simulink model "hybrid_lht_accumulator"  (R2019b)
settings: Solver=FixedStepDiscrete  StartTime=0.0  StopTime=inf  FixedStep=1/150e6  RelTol=1e-3
InitFcn:
  | hybrid_lht_setup;
StopFcn:
  | hybrid_lht_accumulator_compare;
undefined symbols (not defined in the file or in its folder): bt, height, nTheta, width
libraries: hdlsllib x20, simulink x17, dspsrcs4 x1
(part 2 of 2)

== system hybrid_lht_accumulator/Hybrid LHT/Hybrid LHT Accumulator/Accumulator with Switches/Accumulator/Block RAM ==
  wr_data : Inport
  wr_addr : Inport  Port=2
  wr_en : Inport  Port=3
  rd_addr : Inport  Port=4
  Simple Dual Port RAM : Subsystem  VariantControl=9_bits
  Simple Dual Port RAM Generator : Subsystem  VariantControl=other_bits  mask{b=36, d=400, b_hidden=12, d_hidden=2204}
      mask prompts: b "Data width:"; d "Depth:"
      mask init:
      | if b == b_hidden && d == d_hidden
      |     return
      | end
      | 
      | % Xilinx RAM Initialisation
      | xl_config = [512, 72;
      |             1024, 36;
      |             2048, 18;
      |             4096, 9;
      |             8192, 4;
      |             16384, 2;
      |             32768, 1];
      | 
      | % Get length of Xilinx Configuration
      | sizeram = size(xl_config);
      |         
      | % Get the RAM Configuration based on the data width
      | for i = 1:sizeram(1)
      |     if b <= xl_config(i, 2)
      |         a = xl_config(i, :);
      |     end
      | end
      | 
      | % Get number of BRAM required (including half BRAM)
      | numbram = ceil((d/a(1))/0.5)*0.5;
      | fullbram = floor(numbram); % Integer
      | halfbram = (numbram-floor(numbram)) ~= 0; % Boolean
      | 
      | % Get all blocks and delete everything excepts ports
      | H = get(find_system(gcb, 'FindAll', 'on', 'type', 'block'));
      | todelete = setdiff(strcat(repmat({[gcb '/']}, numel(H.Blocks), 1),  H.Blocks),...
      |     strcat(repmat({[gcb '/']}, 5, 1),...
      |     {'wr_data'; 'wr_addr'; 'wr_en'; 'rd_addr'; 'rd_data'}));
      | delete_block(todelete);
      | 
      | % Delete lines
      | for i = 1:numel(H.Lines)
      |     delete_line(H.Lines(i).Handle)
      | end
      | 
      | % Generate full BRAMs
      | y = 0;
      | 
      | % If there is only one ram then the write enable should be directly
      | % connected to the first ram write enable. Else, the write address must be sliced
      | % and the upper bound (over a(2)) compared to zero. This will indicate if
      | % the first ram is the one to be written/read from.
      | 
      | % Common to both implementations
      | % Write Address Slice
      | add_block('hdlsllib/Logic and Bit Operations/Bit Slice',...
      |         [gcb, '/wr_address'], 'Position',...
      |         [160 130 250 170]);
      | % Set bitslice parameters
      | set_param([gcb, '/wr_address'],...
      |     'lidx', int2str(log2(a(1))-1));
      | set_param([gcb, '/wr_address'],...
      |     'ridx', int2str(0));
      | 
      | % Read Address Slice
      | add_block('hdlsllib/Logic and Bit Operations/Bit Slice',...
      |         [gcb, '/rd_address'], 'Position',...
      |         [160 330 250 370]);
      | % Set bitslice parameters
      | set_param([gcb, '/rd_address'],...
      |     'lidx', int2str(log2(a(1))-1));
      | set_param([gcb, '/rd_address'],...
      |     'ridx', int2str(0));
      | 
      | if ceil(numbram) == 1
      |     
      |     i = 1;
      |     
      |     % Add Simple RAM
      |     add_block('hdlsllib/HDL RAMs/Simple Dual Port RAM',...
      |         [gcb, '/simple_ram_', int2str(i-1)], 'Position',...
      |         [635 0+600*y 635+200 400+600*y]);
      | 
      |     % Set RAM parameters
      |     set_param([gcb, '/simple_ram_', int2str(i-1)],...
      |         'ram_size', int2str(log2(a(1))));
      | 
      |     % Connect "wr_data" to "simple_ram_i"
      |     add_line(gcb, ['wr_data/1'], ['simple_ram_', int2str(i-1), '/1'],...
      |         'autorouting', 'on');
      |     
      |     % Connect "wr_addr" to "wr_address"
      |     add_line(gcb, ['wr_addr/1'], ['wr_address/1'],...
      |         'autorouting', 'on');
      | 
      |     % Connect "wr_address" to "simple_ram_i"
      |     add_line(gcb, ['wr_address/1'], ['simple_ram_', int2str(i-1), '/2'],...
      |         'autorouting', 'on');
      | 
      |     % Connect "wr_en" to "simple_ram_i"
      |     add_line(gcb, ['wr_en/1'], ['simple_ram_', int2str(i-1), '/3'],...
      |         'autorouting', 'on');
      |     
      |     % Connect "rd_addr" to "rd_address"
      |     add_line(gcb, ['rd_addr/1'], ['rd_address/1'],...
      |         'autorouting', 'on');
      | 
      |     % Connect "rd_address" to "simple_ram_i"
      |     add_line(gcb, ['rd_address/1'], ['simple_ram_', int2str(i-1), '/4'],...
      |         'autorouting', 'on');
      | 
      |     % Connect "simple_ram_i" to "rd_data"
      |     add_line(gcb, ['simple_ram_', int2str(i-1), '/1'], ['rd_data/1'],...
      |         'autorouting', 'on');
      | 
      | else
      |     
      |     % Multiport Switch
      |     add_block('hdlsllib/Signal Routing/Multiport Switch',...
      |         [gcb, '/multiport_switch'], 'Position',...
      |         [1340 146 1405 250]);
      |     % Set multiport switch parameters
      |     set_param([gcb, '/multiport_switch'],...
      |         'Inputs', int2str(ceil(numbram)));
      |     set_param([gcb, '/multiport_switch'],...
      |         'DataPortOrder', 'Zero-based contiguous');
      | 
      |     % Add Constant Zero
      |     add_block('hdlsllib/Sources/Constant',...
      |         [gcb, '/zero'], 'Position',...
      |         [425 -65 455 -35]);
      |     set_param([gcb, '/zero'],...
      |         'Value', int2str(0));
      |     set_param([gcb, '/zero'],...
      |         'OutDataTypeStr', ['fixdt(0, ', int2str(ceil(numbram)), ', 0)']);
      | 
      |     % Add Vector Concatenate
      |     add_block('hdlsllib/Signal Routing/Vector Concatenate',...
      |         [gcb, '/vector_concatenate'], 'Position',...
      |         [1015, -113, 1025, 38]);
      |     set_param([gcb, '/vector_concatenate'],...
      |         'NumInputs', int2str(ceil(numbram)));
      | 
      |     % Add Bitwise-OR
      |     add_block('hdlsllib/Logic and Bit Operations/Bitwise Operator',...
      |         [gcb, '/bitwise_or'], 'Position',...
      |         [1165, -54, 1205, -16]);
      |     set_param([gcb, '/bitwise_or'],...
      |         'logicop', 'OR');
      |     set_param([gcb, '/bitwise_or'],...
      |         'UseBitMask', 0);
      |     set_param([gcb, '/bitwise_or'],...
      |         'NumInputPorts', int2str(1));
      | 
      |     % Add delay for bram access
      |     add_block('hdlsllib/Discrete/Delay',...
      |         [gcb, '/delay'], 'Position',...
      |         [1248, 60, 1282, 95]);
      |     set_param([gcb, '/delay'],...
      |         'DelayLength', int2str(1));
      |     
      |     % Add bitslice
      |     add_block('hdlsllib/Logic and Bit Operations/Bit Slice',...
      |         [gcb, '/wr_bitslice'], 'Position',...
      |         [-65 180 25 220]);
      | 
      |     % Set bitslice parameters
      |     set_param([gcb, '/wr_bitslice'],...
      |         'lidx', int2str(ceil(log2(d)-1)));
      |     set_param([gcb, '/wr_bitslice'],...
      |         'ridx', int2str(log2(a(1))));
      |     
      |     % Add bitslice
      |     add_block('hdlsllib/Logic and Bit Operations/Bit Slice',...
      |         [gcb, '/rd_bitslice'], 'Position',...
      |         [-65 280 25 320]);
      | 
      |     % Set bitslice parameters
      |     set_param([gcb, '/rd_bitslice'],...
      |         'lidx', int2str(ceil(log2(d)-1)));
      |     set_param([gcb, '/rd_bitslice'],...
      |         'ridx', int2str(log2(a(1))));
      |     
      |     for i = 1:ceil(numbram)
      |         
      |         %%%%% Begin Adding Blocks %%%%%
      |         % Add Simple RAM
      |         add_block('hdlsllib/HDL RAMs/Simple Dual Port RAM',...
      |             [gcb, '/simple_ram_', int2str(i-1)], 'Position',...
      |             [635 0+600*y 635+200 400+600*y]);
      | 
      |         % Set RAM parameters
      |         set_param([gcb, '/simple_ram_', int2str(i-1)],...
      |             'ram_size', int2str(log2(a(1))));
      | 
      |         % Add compare to constant
      |         add_block('hdlsllib/Logic and Bit Operations/Compare To Constant',...
      |             [gcb, '/wr_cmp2const_', int2str(i-1)], 'Position',...
      |             [190 225+y*600 220 255+y*600]); 
      | 
      |         % Set compare to zero parameters
      |         set_param([gcb, '/wr_cmp2const_', int2str(i-1)],...
      |             'relop', '==');
      | 
      |         % Set compare to zero parameters
      |         set_param([gcb, '/wr_cmp2const_', int2str(i-1)],...
      |             'const', int2str(i-1));
      |         
      |         % Add compare to constant
      |         add_block('hdlsllib/Logic and Bit Operations/Compare To Constant',...
      |             [gcb, '/rd_cmp2const_', int2str(i-1)], 'Position',...
      |             [190 445+y*600 220 475+y*600]); 
      | 
      |         % Set compare to zero parameters
      |         set_param([gcb, '/rd_cmp2const_', int2str(i-1)],...
      |             'relop', '==');
      | 
      |         % Set compare to zero parameters
      |         set_param([gcb, '/rd_cmp2const_', int2str(i-1)],...
      |             'const', int2str(i-1));
      | 
      |         % Add and logic
      |         add_block('hdlsllib/Logic and Bit Operations/Logical Operator',...
      |             [gcb, '/and_', int2str(i-1)], 'Position',...
      |             [420 231+600*y 455 264+600*y]);
      | 
      |         % Set and logic parameters
      |         set_param([gcb, '/and_', int2str(i-1)],...
      |             'Operator', 'AND');
      | 
      |         % Add Switch
      |         add_block('hdlsllib/Signal Routing/Switch',...
      |             [gcb, '/switch_', int2str(i-1)], 'Position',...
      |             [685 -113+600*y 785 -37+600*y]);
      | 
      |         % Set switch parameters
      |         set_param([gcb, '/switch_', int2str(i-1)],...
      |             'Threshold', int2str(1));
      | 
      |         % Add Constant
      |         add_block('hdlsllib/Sources/Constant',...
      |             [gcb, '/constant_', int2str(i-1)], 'Position',...
      |             [425 -115+600*y 455 -85+600*y]);
      | 
      |         % Set Constant parameters
      |         set_param([gcb, '/constant_', int2str(i-1)],...
      |             'Value', int2str(i-1));
      |         set_param([gcb, '/constant_', int2str(i-1)],...
      |             'OutDataTypeStr', ['fixdt(0, ', int2str(ceil(numbram)), ', 0)']);   
      | 
      |         %%%%% Begin Wire Connections %%%%%        
      |         % Connect "wr_data" to "simple_ram_i"
      |         add_line(gcb, 'wr_data/1', ['simple_ram_', int2str(i-1), '/1'],...
      |             'autorouting','on');
      | 
      |         % Connect "wr_address" to "simple_ram_i"
      |         add_line(gcb, 'wr_address/1', ['simple_ram_', int2str(i-1), '/2'],...
      |             'autorouting','on');
      | 
      |         % Connect "rd_address" to "simple_ram_i"
      |         add_line(gcb, 'rd_address/1', ['simple_ram_', int2str(i-1), '/4'],...
      |             'autorouting','on');
      | 
      |         % Connect "constant_i" to "switch_i"
      |         add_line(gcb, ['constant_', int2str(i-1), '/1'], ['switch_', int2str(i-1), '/1'],...
      |             'autorouting','on');
      | 
      |         % Connect "zero" to "switch_i"
      |         add_line(gcb, 'zero/1', ['switch_', int2str(i-1), '/3'],...
      |             'autorouting','on');
      | 
      |         % Connect "switch_i" to "vector_concatenate"
      |         add_line(gcb, ['switch_', int2str(i-1), '/1'], ['vector_concatenate/', int2str(i)],...
      |             'autorouting','on');
      | 
      |         % Connect "rd_address" to "simple_ram_i"
      |         add_line(gcb, ['simple_ram_', int2str(i-1), '/1'],['multiport_switch/', int2str(i+1)],...
      |             'autorouting','on');
      | 
      |         % Connect "bitslice_i" to "wr_cmp2const_i"
      |         add_line(gcb, ['wr_bitslice/1'], ['wr_cmp2const_', int2str(i-1), '/1'],...
      |             'autorouting','on');
      |         
      |         % Connect "bitslice_i" to "rd_cmp2const_i"
      |         add_line(gcb, ['rd_bitslice/1'], ['rd_cmp2const_', int2str(i-1), '/1'],...
      |             'autorouting','on');
      | 
      |         % Connect "wr_en" to "and_i"
      |         add_line(gcb, ['wr_en/1'], ['and_', int2str(i-1), '/2'],...
      |             'autorouting','on');
      | 
      |         % Connect "and_i" to "simple_ram_0"
      |         add_line(gcb, ['and_', int2str(i-1), '/1'], ['simple_ram_', int2str(i-1), '/3'],...
      |             'autorouting','on');
      | 
      |         % Connect "wr_cmp2const_i" to "and_i"
      |         add_line(gcb, ['wr_cmp2const_', int2str(i-1), '/1'], ['and_', int2str(i-1), '/1'],...
      |             'autorouting','on');
      | 
      |         % Connect "rd_cmp2const_i" to "switch_i"
      |         add_line(gcb, ['rd_cmp2const_', int2str(i-1), '/1'], ['switch_', int2str(i-1), '/2'],...
      |             'autorouting','on');
      |          
      |         % Update coordinates
      |         y = y + 1;
      |         
      |     end
      |     
      |     % Connect "rd_addr" to "bitslice_i"
      |     add_line(gcb, ['rd_addr/1'], ['rd_bitslice/1'],...
      |         'autorouting','on');
      |     
      |     % Connect "wr_addr" to "bitslice_i"
      |     add_line(gcb, ['wr_addr/1'], ['wr_bitslice/1'],...
      |         'autorouting','on');
      |     
      |     % Connect "wr_addr" to "wr_address"
      |     add_line(gcb, 'wr_addr/1', ['wr_address', '/1'],...
      |         'autorouting','on');
      | 
      |     % Connect "rd_addr" to "rd_address"
      |     add_line(gcb, 'rd_addr/1', ['rd_address', '/1'],...
      |         'autorouting','on');
      | 
      |     % Connect "vector_concatenate" to "bitwise_or"
      |     add_line(gcb, ['vector_concatenate/1'], ['bitwise_or/1'],...
      |         'autorouting','on');
      | 
      |     % Connect "bitwise_or" to "delay"
      |     add_line(gcb, ['bitwise_or/1'], ['delay/1'],...
      |         'autorouting','on');
      | 
      |     % Connect "delay" to "multiport_switch"
      |     add_line(gcb, ['delay/1'], ['multiport_switch/1'],...
      |         'autorouting','on');
      | 
      |     % Connect "multiport_switch" to "rd_data"
      |     add_line(gcb, ['multiport_switch/1'], ['rd_data/1'],...
      |         'autorouting','on');
      |     
      | end
      | 
      | % If there is a half bram we must change a few parameters. Firstly, delete
      | % the write and read address lines. Then add bitslice blocks to reduce the
      | % address space in half. Connect rd_addr and wr_addr to the corresponding ports
      | % on the bram. Finally, change the address depth.
      | if halfbram
      |     
      |     if ceil(numbram) > 1
      |         
      |         % Delete lines
      |         delete_line(gcb, ['wr_address/1'], ['simple_ram_', int2str(i-1), '/2'])
      |         delete_line(gcb, ['rd_address/1'], ['simple_ram_', int2str(i-1), '/4'])
      |         
      |         % Write Address half ram Slice
      |         add_block('hdlsllib/Logic and Bit Operations/Bit Slice',...
      |                 [gcb, '/wr_address_hr'], 'Position',...
      |                 [160 130+(y-1)*600 250 170+(y-1)*600]);
      |         % Set bitslice parameters
      |         set_param([gcb, '/wr_address_hr'],...
      |             'lidx', int2str(log2(a(1))-2));
      |         set_param([gcb, '/wr_address_hr'],...
      |             'ridx', int2str(0));
      | 
      |         % Read Address half ram Slice
      |         add_block('hdlsllib/Logic and Bit Operations/Bit Slice',...
      |                 [gcb, '/rd_address_hr'], 'Position',...
      |                 [160 330+(y-1)*600 250 370+(y-1)*600]);
      |         % Set bitslice parameters
      |         set_param([gcb, '/rd_address_hr'],...
      |             'lidx', int2str(log2(a(1))-2));
      |         set_param([gcb, '/rd_address_hr'],...
      |             'ridx', int2str(0));
      | 
      |         % Connect "wr_addr" to "wr_address_hr"
      |         add_line(gcb, 'wr_addr/1', ['wr_address_hr', '/1'],...
      |             'autorouting','on');
      | 
      |         % Connect "rd_addr" to "rd_address_hr"
      |         add_line(gcb, 'rd_addr/1', ['rd_address_hr', '/1'],...
      |             'autorouting','on');
      | 
      |         % Connect "wr_address_hr" to "simple_ram_i"
      |         add_line(gcb, ['wr_address_hr', '/1'], ['simple_ram_', int2str(i-1), '/2'],...
      |             'autorouting','on');
      | 
      |         % Connect "rd_address_hr" to "simple_ram_i"
      |         add_line(gcb, ['rd_address_hr', '/1'], ['simple_ram_', int2str(i-1), '/4'],...
      |             'autorouting','on');
      | 
      |     else
      |         % Set bitslice parameters
      |         set_param([gcb, '/wr_address'],...
      |             'lidx', int2str(log2(a(1))-2));
      |         set_param([gcb, '/wr_address'],...
      |             'ridx', int2str(0));
      |         % Set bitslice parameters
      |         set_param([gcb, '/rd_address'],...
      |             'lidx', int2str(log2(a(1))-2));
      |         set_param([gcb, '/rd_address'],...
      |             'ridx', int2str(0));
      |         
      |     end
      |     
      |     % Update the ram parameters (address bits)
      |     set_param([gcb, '/simple_ram_', int2str(i-1)],...
      |         'ram_size', int2str(log2(a(1)/2)));
      |     
      | end
      | 
      | b_hidden = b;
      | d_hiddne = d;
  rd_data : Outport

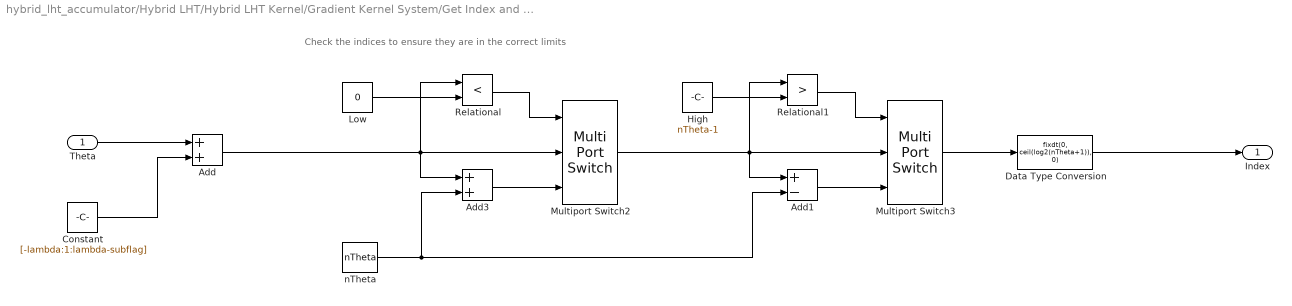
== system hybrid_lht_accumulator/Hybrid LHT/Hybrid LHT Kernel/Gradient Kernel System/Get Index and Fix Limits/Extract Active Votes ==
  note: Check the indices to ensure they are in the correct limits
  Theta : Inport
  Add : Sum
  Add1 : Sum  Inputs=+-
  Add3 : Sum
  Constant : Constant  Value=[-lambda:1:lambda-subflag]  VectorParams1D=off  OutDataTypeStr=fixdt(1,ceil(log2(lambda+1))+1, 0)  SampleTime=-1
  Data Type Conversion : DataTypeConversion  OutDataTypeStr=fixdt(0, ceil(log2(nTheta+1)), 0)
  High : Constant  Value=nTheta-1  OutDataTypeStr=fixdt(0,ceil(log2(nTheta)),0)  SampleTime=-1
  Low : Constant  Value=0  OutDataTypeStr=fixdt(0,1,0)  SampleTime=-1
  Multiport Switch2 : MultiPortSwitch  DataPortOrder=Zero-based contiguous  Inputs=2  zeroidx=on
  Multiport Switch3 : MultiPortSwitch  DataPortOrder=Zero-based contiguous  Inputs=2  zeroidx=on
  Relational : RelationalOperator  Operator=<  OutDataTypeStr=boolean  RndMeth=Nearest
  Relational1 : RelationalOperator  Operator=>  OutDataTypeStr=boolean  RndMeth=Nearest
  nTheta : Constant  Value=nTheta  OutDataTypeStr=fixdt(0,ceil(log2(nTheta+1)),0)  SampleTime=-1
  Index : Outport  VectorParamsAs1DForOutWhenUnconnected=off
  wires:
  Constant/1 -> Add/2
  Add1/1 -> Multiport Switch3/3
  Relational/1 -> Multiport Switch2/1
  Multiport Switch3/1 -> Data Type Conversion/1
  High/1 -> Relational1/2
  Relational1/1 -> Multiport Switch3/1
  Add3/1 -> Multiport Switch2/3
  Low/1 -> Relational/2
  Multiport Switch2/1 -> Add1/1, Relational1/1, Multiport Switch3/2
  nTheta/1 -> Add3/2, Add1/2
  Add/1 -> Add3/1, Relational/1, Multiport Switch2/2
  Theta/1 -> Add/1
  Data Type Conversion/1 -> Index/1

== system hybrid_lht_accumulator/Hybrid LHT/Hybrid LHT Kernel/Gradient Kernel System/Get Index and Fix Limits/GetShift1 ==
  Theta : Inport  Partition=on  PartitionDimension=2  PartitionWidth=1  PartitionOffset=0
  Add : Sum  Inputs=+  OutDataTypeStr=fixdt(0, ceil(log2(L+1)), 0)
  Constant : Constant  Value=U  VectorParams1D=off  OutDataTypeStr=fixdt(0,ceil(log2(max(U)+1)),0)  SampleTime=-1
  For Each : ForEach  DisableCoverage=on
  Relational Operator : RelationalOperator  OutDataTypeStr=boolean  RndMeth=Nearest
  Shift : Outport  ConcatenationDimension=2  VectorParamsAs1DForOutWhenUnconnected=off
  wires:
  Constant/1 -> Relational Operator/2
  Theta/1 -> Relational Operator/1
  Add/1 -> Shift/1
  Relational Operator/1 -> Add/1

== system hybrid_lht_accumulator/Hybrid LHT/Hybrid LHT Kernel/Gradient Kernel System/Hough Kernel/Hough Kernel ==
  X : Inport
  Y : Inport  Port=2
  Index : Inport  Port=3
  Add : Sum  OutDataTypeStr=fixdt(1, ceil(log2(2*maxRho)), 0)  RndMeth=Round
  CosineROM : Constant  Value=fi(cos(deg2rad(theta)), 1, 16, 14)  VectorParams1D=off  OutDataTypeStr=fixdt(1,16,14)  SampleTime=-1
  Selector : Selector  NumberOfDimensions=2  IndexMode=Zero-based  InputPortWidth=3  IndexOptions=Index vector (dialog),Index vector (port)  Indices=0,1  OutputSizes=1,1
  Selector1 : Selector  NumberOfDimensions=2  IndexMode=Zero-based  InputPortWidth=3  IndexOptions=Index vector (dialog),Index vector (port)  Indices=0,1  OutputSizes=1,1
  xcos : Product  OutDataTypeStr=fixdt(1, ceil(log2(width+1)), 0);  RndMeth=Round
  Rho : Outport  VectorParamsAs1DForOutWhenUnconnected=off
  wires:
  Index/1 -> Selector1/2, Selector/2
  X/1 -> xcos/1
  Selector1/1 -> Add/2
  Add/1 -> Rho/1
  xcos/1 -> Add/1
  Selector/1 -> xcos/2
  CosineROM/1 -> Selector/1
  Y/1 -> Selector1/1

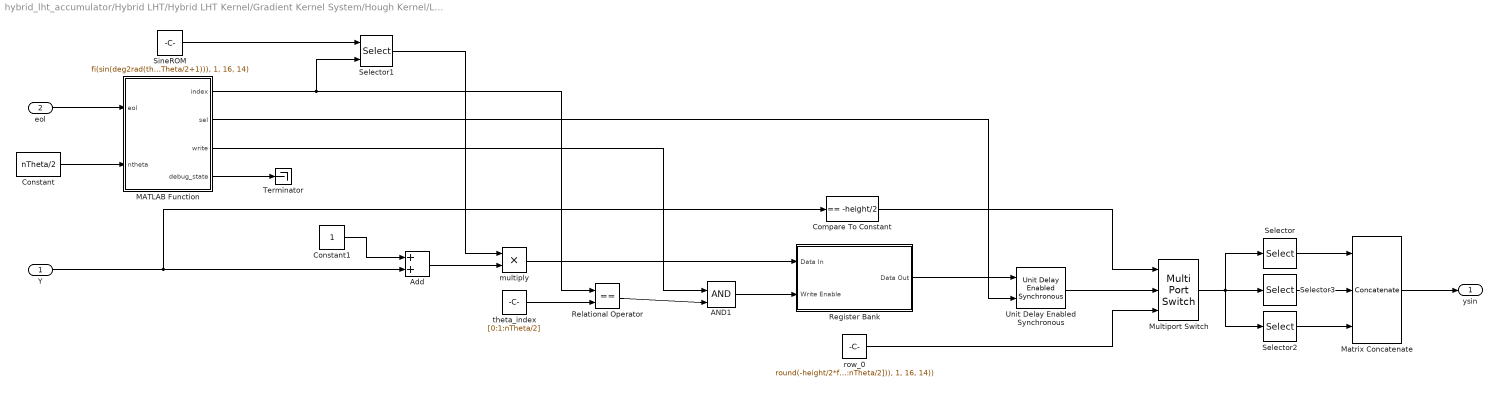
== system hybrid_lht_accumulator/Hybrid LHT/Hybrid LHT Kernel/Gradient Kernel System/Hough Kernel/Look Ahead Hough ==
  Y : Inport
  eol : Inport  Port=2
  AND1 : Logic  IconShape=distinctive  AllPortsSameDT=off  OutDataTypeStr=boolean
  Add : Sum  OutDataTypeStr=fixdt(1,ceil(log2(height)),0)
  Compare To Constant : simulink/Logic and Bit Operations/Compare To Constant  relop===  const=-height/2  OutDataTypeStr=boolean
  Constant : Constant  Value=nTheta/2  OutDataTypeStr=fixdt(0, ceil(log2(nTheta+1)), 0)  SampleTime=-1
  Constant1 : Constant  OutDataTypeStr=fixdt(1, ceil(log2(height)), 0);  SampleTime=-1
  MATLAB Function : MATLAB Function  TreatAsAtomicUnit=on
  Matrix Concatenate : Concatenate  NumInputs=3  Mode=Multidimensional array  ConcatenateDimension=2
  Multiport Switch : MultiPortSwitch  DataPortOrder=Zero-based contiguous  Inputs=2  zeroidx=on
  Register Bank : Subsystem  TreatAsAtomicUnit=on
  Relational Operator : RelationalOperator  Operator===  OutDataTypeStr=boolean  RndMeth=Simplest
  Selector : Selector  NumberOfDimensions=2  IndexMode=Zero-based  InputPortWidth=3  IndexOptions=Index vector (dialog),Index vector (dialog)  Indices=0,[0:1:nTheta/2-1]  OutputSizes=1,1
  Selector1 : Selector  NumberOfDimensions=2  IndexMode=Zero-based  InputPortWidth=3  IndexOptions=Index vector (dialog),Index vector (port)  Indices=0,1  OutputSizes=1,1
  Selector2 : Selector  NumberOfDimensions=2  IndexMode=Zero-based  InputPortWidth=3  IndexOptions=Index vector (dialog),Index vector (dialog)  Indices=0,[nTheta/2-1:-1:1]  OutputSizes=1,1
  Selector3 : Selector  NumberOfDimensions=2  IndexMode=Zero-based  InputPortWidth=3  IndexOptions=Index vector (dialog),Index vector (dialog)  Indices=0,nTheta/2  OutputSizes=1,1
  SineROM : Constant  Value=fi(sin(deg2rad(theta(1:1:nTheta/2+1))), 1, 16, 14)  VectorParams1D=off  OutDataTypeStr=fixdt(1,16,14)  SampleTime=-1
  Terminator : Terminator
  Unit Delay Enabled Synchronous : hdlsllib/Discrete/Unit Delay Enabled Synchronous  InitialCondition=0.0  SampleTime=-1
      settings: SourceProductName=Simulink  SourceProductBaseCode=SL
  multiply : Product  OutDataTypeStr=fixdt(1, ceil(log2(height)), 0);  RndMeth=Round
  row_0 : Constant  Value=round(-height/2*fi(sin(deg2rad([0:1:nTheta/2])), 1, 16, 14))  VectorParams1D=off  OutDataTypeStr=fixdt(1,ceil(log2(height)),0)  SampleTime=-1
  theta_index : Constant  Value=[0:1:nTheta/2]  VectorParams1D=off  OutDataTypeStr=fixdt(0,ceil(log2(max(theta)+1)),0)  SampleTime=-1
  ysin : Outport  VectorParamsAs1DForOutWhenUnconnected=off
  wires:
  Multiport Switch/1 -> Selector2/1, Selector3/1, Selector/1
  Unit Delay Enabled Synchronous/1 -> Multiport Switch/2
  Register Bank/1(Data Out) -> Unit Delay Enabled Synchronous/1
  Compare To Constant/1 -> Multiport Switch/1
  MATLAB Function/2(sel) -> Unit Delay Enabled Synchronous/2
  SineROM/1 -> Selector1/1
  Matrix Concatenate/1 -> ysin/1
  Selector3/1 -> Matrix Concatenate/2
  Selector/1 -> Matrix Concatenate/1
  MATLAB Function/4(debug_state) -> Terminator/1
  AND1/1 -> Register Bank/2(Write Enable)
  Relational Operator/1 -> AND1/2
  theta_index/1 -> Relational Operator/2
  multiply/1 -> Register Bank/1(Data In)
  Selector1/1 -> multiply/1
  MATLAB Function/1(index) -> Relational Operator/1, Selector1/2
  eol/1 -> MATLAB Function/1(eol)
  Constant/1 -> MATLAB Function/2(ntheta)
  MATLAB Function/3(write) -> AND1/1
  Constant1/1 -> Add/1
  Y/1 -> Compare To Constant/1, Add/2
  Add/1 -> multiply/2
  row_0/1 -> Multiport Switch/3
  Selector2/1 -> Matrix Concatenate/3

== system hybrid_lht_accumulator/Hybrid LHT/Hybrid LHT Accumulator/Accumulator with Switches/Accumulator/Block RAM/Simple Dual Port RAM ==
  wr_data : Inport
  wr_addr : Inport  Port=2
  wr_en : Inport  Port=3
  rd_addr : Inport  Port=4
  Simple Dual Port RAM : hdlsllib/HDL RAMs/Simple Dual Port RAM  ram_size=ceil(log2(maxRho*2))
      settings: SourceProductName=Simulink  SourceProductBaseCode=SL
  rd_data : Outport
  wires:
  Simple Dual Port RAM/1 -> rd_data/1
  rd_addr/1 -> Simple Dual Port RAM/4
  wr_en/1 -> Simple Dual Port RAM/3
  wr_addr/1 -> Simple Dual Port RAM/2
  wr_data/1 -> Simple Dual Port RAM/1

== system hybrid_lht_accumulator/Hybrid LHT/Hybrid LHT Accumulator/Accumulator with Switches/Accumulator/Block RAM/Simple Dual Port RAM Generator ==
  wr_data : Inport
  wr_addr : Inport  Port=2
  wr_en : Inport  Port=3
  rd_addr : Inport  Port=4
  rd_address : hdlsllib/Logic and Bit Operations/Bit Slice  lidx=8  ridx=0
      settings: SourceProductName=Simulink  SourceProductBaseCode=SL
  simple_ram_0 : hdlsllib/HDL RAMs/Simple Dual Port RAM  ram_size=9
      settings: SourceProductName=Simulink  SourceProductBaseCode=SL
  wr_address : hdlsllib/Logic and Bit Operations/Bit Slice  lidx=8  ridx=0
      settings: SourceProductName=Simulink  SourceProductBaseCode=SL
  rd_data : Outport
  wires:
  wr_data/1 -> simple_ram_0/1
  wr_addr/1 -> wr_address/1
  wr_address/1 -> simple_ram_0/2
  wr_en/1 -> simple_ram_0/3
  rd_addr/1 -> rd_address/1
  rd_address/1 -> simple_ram_0/4
  simple_ram_0/1 -> rd_data/1

== system hybrid_lht_accumulator/Hybrid LHT/Hybrid LHT Kernel/Gradient Kernel System/Hough Kernel/Look Ahead Hough/Register Bank ==
  Data In : Inport
  Write Enable : Inport  Port=2  Partition=on  PartitionDimension=2  PartitionWidth=1  PartitionOffset=0
  For Each : ForEach  DisableCoverage=on
  Unit Delay Enabled Synchronous : hdlsllib/Discrete/Unit Delay Enabled Synchronous  InitialCondition=0.0  SampleTime=-1
      settings: SourceProductName=Simulink  SourceProductBaseCode=SL
  Data Out : Outport  ConcatenationDimension=2
  wires:
  Data In/1 -> Unit Delay Enabled Synchronous/1
  Unit Delay Enabled Synchronous/1 -> Data Out/1
  Write Enable/1 -> Unit Delay Enabled Synchronous/2

== matlab function hybrid_lht_accumulator/Hybrid LHT/Hybrid LHT Accumulator/Accumulator Controller ==
  data: shift output; sof input; mode output; eof input; read output; clear output; index output; ntheta input; nrho input; valid output; nshift input
function [shift, mode, read, clear, index, valid] = fcn(sof, eof, ntheta, nrho, nshift)

IDLE = fi(0, 0, 2, 0);
VOTE = fi(1, 0, 2, 0);
READ = fi(2, 0, 2, 0);
CLEAR = fi(3, 0, 2, 0);

persistent current_state;
persistent rho_counter;
persistent theta_counter;
persistent shift_counter;

if isempty(current_state)
    current_state = IDLE;
end

if isempty(rho_counter)
    rho_counter = fi(0, 0, 16, 0);
end

if isempty(theta_counter)
    theta_counter = fi(0, 0, 16, 0);
end

if isempty(shift_counter)
    shift_counter = fi(0, 0, 16, 0);
end

switch current_state
    case IDLE
        rho_counter = fi(0, 0, 16, 0);
        theta_counter = fi(0, 0, 16, 0);
        shift_counter = fi(0, 0, 16, 0);
        
        clear = false;
        valid = false;
        
        read = rho_counter;
        index = theta_counter;
        shift = shift_counter;
        
        if sof
            mode = true;
            current_state = VOTE;
        else
            mode = false;
            current_state = IDLE;
        end
        
    case VOTE
        rho_counter = fi(0, 0, 16, 0);
        theta_counter = fi(0, 0, 16, 0);
        shift_counter = fi(0, 0, 16, 0);
        
        mode = true;
        clear = false;
        valid = false;
        
        shift = shift_counter;
        read = rho_counter;
        index = theta_counter;
        
        if eof
            current_state = READ;
        else
            current_state = VOTE;
        end
        
    case READ
        mode = false;
        clear = false;
        valid = true;
        
        read = rho_counter;
        index = theta_counter;
        shift = shift_counter;
        
        if theta_counter >= ntheta && rho_counter >= nrho && shift_counter >= nshift
            rho_counter = fi(0, 0, 16, 0);
            theta_counter = fi(0, 0, 16, 0);
            shift_counter = fi(0, 0, 16, 0);
            current_state = CLEAR;
        elseif theta_counter >= ntheta && rho_counter >= nrho
            theta_counter = fi(0, 0, 16, 0);
            rho_counter = fi(0, 0, 16, 0);
            shift_counter = fi(shift_counter + 1, 0, 16, 0);
            current_state = READ;
        elseif rho_counter >= nrho
            rho_counter = fi(0, 0, 16, 0);
            theta_counter = fi(theta_counter + 1, 0, 16, 0);
            current_state = READ;
        else
            rho_counter = fi(rho_counter + 1, 0, 16, 0);
            current_state = READ;
        end
        
    case CLEAR
        mode = false;
        clear = true;
        valid = false;
        
        read = rho_counter;
        index = theta_counter;
        shift = shift_counter;
        
        if rho_counter >= nrho
            rho_counter = fi(0, 0, 16, 0);
            theta_counter = fi(0, 0, 16, 0);
            shift_counter = fi(0, 0, 16, 0);
            current_state = IDLE;
        else
            rho_counter = fi(rho_counter + 1, 0, 16, 0);
            theta_counter = fi(0, 0, 16, 0);
            shift_counter = fi(0, 0, 16, 0);
            current_state = CLEAR;
        end
        
    otherwise
        rho_counter = fi(0, 0, 16, 0);
        theta_counter = fi(0, 0, 16, 0);
        shift_counter = fi(0, 0, 16, 0);
        
        mode = false;
        clear = false;
        valid = false;
        
        shift = shift_counter;
        read = rho_counter;
        index = theta_counter;
        
        current_state = IDLE;
        
end

== matlab function hybrid_lht_accumulator/Hybrid LHT/Hybrid LHT Kernel/Gradient Kernel System/Hough Kernel/Look Ahead Hough/MATLAB Function ==
  data: index output; eol input; sel output; write output; ntheta input; debug_state output
function [index, sel, write, debug_state] = fcn(eol, ntheta)

BANK = fi(1, 0, 3, 0);
WAIT = fi(2, 0, 3, 0);

persistent state;

persistent thetacounter;

if isempty(state)
    state = BANK;
end

if isempty(thetacounter)
    thetacounter = fi(0, 0, 16, 0);
end

switch state
    case BANK
        sel = false;
        write = true;
        index = thetacounter;
        debug_state = state;
        
        if thetacounter == ntheta
            thetacounter = fi(0, 0, 16, 0);
            state = WAIT;
        else
            thetacounter = fi(thetacounter + 1, 0, 16, 0);
            state = BANK;
        end
        
    case WAIT
        write = false;
        index = thetacounter;
        debug_state = state;
        
        thetacounter = fi(0, 0, 16, 0);
        
        if eol
            sel = true;
            state = BANK;
        else
            sel = false;
            state = WAIT;
        end
        
    otherwise
        thetacounter = fi(0, 0, 16, 0);
        sel = false;
        write = false;
        index = thetacounter;
        debug_state = state;
        
        state = WAIT;
        
end
